simulink model "Projekt_KUS_cyfro_sim"  (R2017a)
settings: Solver=ode45  StartTime=0.0  StopTime=10.0  RelTol=1e-3
undefined symbols (not defined in the file): J, K1, K1I, K2, K2I, Kp, Kt, Mn, omegan, przelacz3, psien, R, T, Top, Tp, Un, Uz0, Y
settings Model: Creator=user  LastModifiedBy=a
settings DataIOCC: LimitDataPoints=on  SaveFormat=Array  SignalLoggingSaveFormat=ModelDataLogs
settings OptimizationCC: BlockReduction=off  BooleanDataType=off  LifeSpan=inf
settings DebuggingCC: SaveWithParameterizedLinksMsg=none  UnderspecifiedInitializationDetection=Classic  MergeDetectMultiDrivingBlocksExec=none  SignalResolutionControl=TryResolveAllWithWarning  MultiTaskDSMMsg=warning  MultiTaskCondExecSysMsg=none  StateNameClashWarn=warning  StrictBusMsg=None  SFUnexpectedBacktrackingDiag=warning  SFNoUnconditionalDefaultTransitionDiag=warning  SFExecutionAtInitializationDiag=none
settings HardwareCC: ProdBitPerPointer=32  ProdBitPerSizeT=32  ProdBitPerPtrDiffT=32  ProdLargestAtomicFloat=None  ProdIntDivRoundTo=Undefined  ProdEndianess=Unspecified  ProdWordSize=32  ProdHWDeviceType=32-bit Generic  TargetUnknown=on
settings ModelReferenceCC: PropagateSignalLabelsOutOfModel=off
settings GRTTargetCC: TargetLangStandard=C89/C90 (ANSI)  GeneratePreprocessorConditionals=Disable all
settings ConfigComp: CovMetricSettings=dw  CovHtmlReporting=on  CovSaveCumulativeToWorkspaceVar=on  CovSaveSingleToWorkspaceVar=on  CovExternalEMLEnable=off

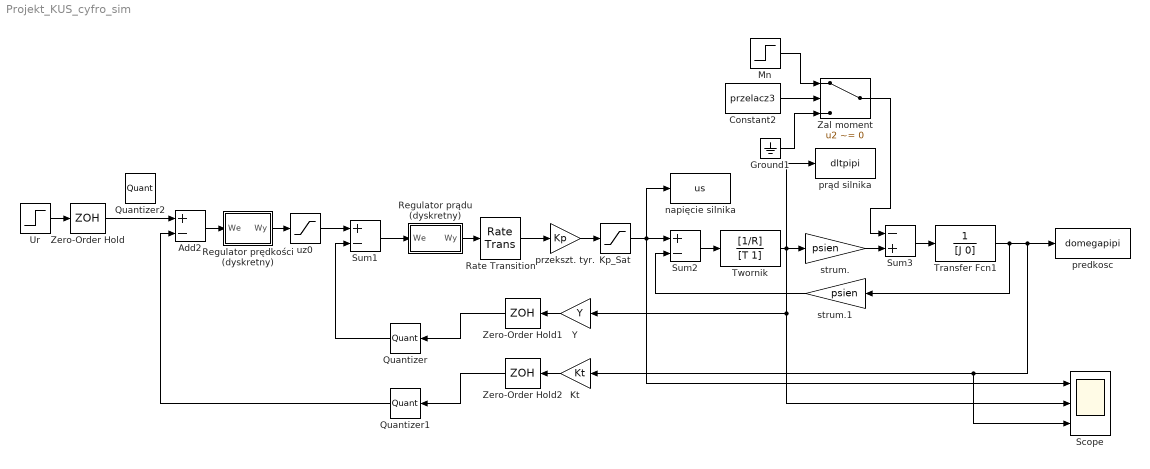
== system Projekt_KUS_cyfro_sim ==
  Add2 : Sum  Inputs=+-
  Constant2 : Constant  Value=przelacz3
  Ground1 : Ground
  Kp_Sat : Saturate  UpperLimit=1.5*Un  LowerLimit=-1.5*Un
  Kt : Gain  Gain=Kt
  Mn : Step  Time=Top  After=Mn  SampleTime=0
  Quantizer : Quantizer  QuantizationInterval=1.1*Tp
  Quantizer1 : Quantizer  QuantizationInterval=1.1*Tp
  Quantizer2 : Quantizer  QuantizationInterval=1.1*Tp
  Rate Transition : RateTransition
  Regulator prądu (dyskretny) : Subsystem
  Regulator prędkości (dyskretny) : Subsystem
  Scope : Scope  NumInputPorts=3
  Sum1 : Sum  Inputs=+-
  Sum2 : Sum  Inputs=+-
  Sum3 : Sum  Inputs=-+
  Transfer Fcn1 : TransferFcn  Denominator=[J 0]
  Twornik : TransferFcn  Numerator=[1/R]  Denominator=[T 1]
  Ur : Step  Time=0  After=Kt*omegan  SampleTime=0
  Y : Gain  Gain=Y
  Zal moment : Switch  Criteria=u2 ~= 0
  Zero-Order Hold : ZeroOrderHold  SampleTime=Tp
  Zero-Order Hold1 : ZeroOrderHold  SampleTime=Tp
  Zero-Order Hold2 : ZeroOrderHold  SampleTime=Tp
  napięcie silnika : ToWorkspace  VariableName=us  SaveFormat=Structure With Time  SampleTime=-1
  predkosc : ToWorkspace  VariableName=domegapipi  SaveFormat=Structure With Time  SampleTime=-1
  przekszt. tyr. : Gain  Gain=Kp
  prąd silnika : ToWorkspace  VariableName=dltpipi  SaveFormat=Structure With Time  SampleTime=-1
  strum. : Gain  Gain=psien
  strum.1 : Gain  Gain=psien
  uz0 : Saturate  UpperLimit=Uz0  LowerLimit=-Uz0
  wires:
  przekszt. tyr./1 -> Kp_Sat/1
  Kp_Sat/1 -> Scope/1, napięcie silnika/1, Sum2/1
  Sum2/1 -> Twornik/1
  Twornik/1 -> prąd silnika/1, Scope/2, Y/1, strum./1
  strum./1 -> Sum3/2
  Sum3/1 -> Transfer Fcn1/1
  Y/1 -> Zero-Order Hold1/1
  Kt/1 -> Zero-Order Hold2/1
  Add2/1 -> Regulator prędkości (dyskretny)/1(We)
  Regulator prędkości (dyskretny)/1(Wy) -> uz0/1
  uz0/1 -> Sum1/1
  Sum1/1 -> Regulator prądu (dyskretny)/1(We)
  Regulator prądu (dyskretny)/1(Wy) -> Rate Transition/1
  Rate Transition/1 -> przekszt. tyr./1
  strum.1/1 -> Sum2/2
  Transfer Fcn1/1 -> Scope/3, Kt/1, predkosc/1, strum.1/1
  Ur/1 -> Zero-Order Hold/1
  Mn/1 -> Zal moment/1
  Zal moment/1 -> Sum3/1
  Constant2/1 -> Zal moment/2
  Ground1/1 -> Zal moment/3
  Zero-Order Hold/1 -> Add2/1
  Zero-Order Hold1/1 -> Quantizer/1
  Quantizer/1 -> Sum1/2
  Quantizer1/1 -> Add2/2
  Zero-Order Hold2/1 -> Quantizer1/1

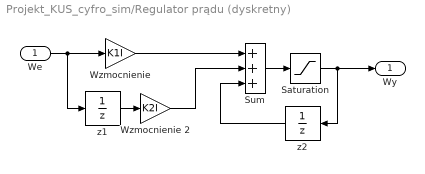
== system Projekt_KUS_cyfro_sim/Regulator prądu (dyskretny) ==
  We : Inport
  Saturation : Saturate  UpperLimit=10  LowerLimit=-10
  Sum : Sum  Inputs=+++
  Wzmocnienie : Gain  Gain=K1I
  Wzmocnienie 2 : Gain  Gain=K2I
  z1 : UnitDelay  SampleTime=Tp
  z2 : UnitDelay  SampleTime=Tp
  Wy : Outport
  wires:
  We/1 -> z1/1, Wzmocnienie/1
  z2/1 -> Sum/3
  Wzmocnienie/1 -> Sum/1
  Sum/1 -> Saturation/1
  Wzmocnienie 2/1 -> Sum/2
  z1/1 -> Wzmocnienie 2/1
  Saturation/1 -> Wy/1, z2/1

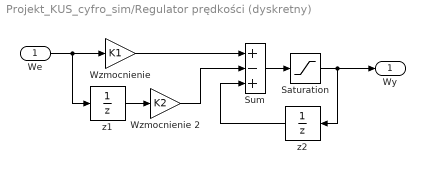
== system Projekt_KUS_cyfro_sim/Regulator prędkości (dyskretny) ==
  We : Inport
  Saturation : Saturate  UpperLimit=10  LowerLimit=-10
  Sum : Sum  Inputs=+-+
  Wzmocnienie : Gain  Gain=K1
  Wzmocnienie 2 : Gain  Gain=K2
  z1 : UnitDelay  SampleTime=Tp
  z2 : UnitDelay  SampleTime=Tp
  Wy : Outport
  wires:
  We/1 -> z1/1, Wzmocnienie/1
  z2/1 -> Sum/3
  Wzmocnienie/1 -> Sum/1
  Sum/1 -> Saturation/1
  Wzmocnienie 2/1 -> Sum/2
  z1/1 -> Wzmocnienie 2/1
  Saturation/1 -> Wy/1, z2/1
